simulink model "simulation model"  (R2022b)
settings: Solver=VariableStepAuto  StartTime=0.0  StopTime=2  RelTol=1e-3
undefined symbols (not defined in the file): a_prop, ACCtime, alfa, alfaPRO, Ba, Bf, Bp, Bv, IPR, matrixA, Ng_safe, No_perf, No_safe, Np, Np_safe, optimal_rotation, P3tDIVP2t_perf, P3tDIVP2t_safe, Q, Q_safe, T45_perf, T45_safe, Wf, xfuel, xlin, y, Yangle
libraries: fl_lib x31, nesl_utility x15, sh_lib x14, simulink x7, slpidlib x4, SimscapeFluids_lib x3
(part 2 of 2)

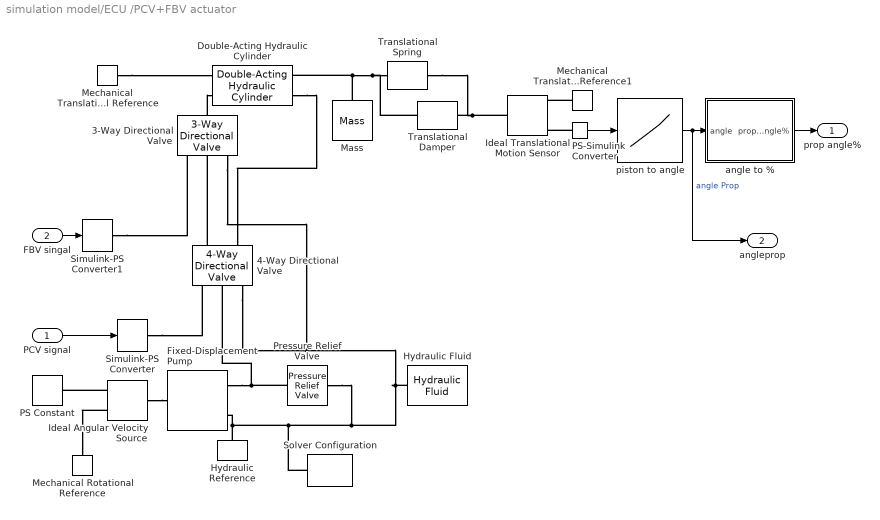
== system simulation model/ECU /PCV+FBV actuator ==
  PCV signal : Inport
  FBV singal : Inport  Port=2
  3-Way Directional Valve : sh_lib/Valves/Directional Valves/3-Way Directional Valve  area_spec=sh.valves.directional_valves.enum.area_spec.identical  mdl_type_identical=sh.valves.directional_valves.enum.mdl_type.linear  mdl_type_different=sh.valves.directional_valves.enum.mdl_type.linear  interp_method_identical=sh.valves.directional_valves.enum.interp_method.linear  interp_method_different=sh.valves.directional_valves.enum.interp_method.linear  extrap_method_identical=sh.valves.directional_valves.enum.extrap_method.linear  extrap_method_different=sh.valves.directional_valves.enum.extrap_method.linear  A_leak=1e-12 m^2  C_d=0.7  lam_spec=sh.valves.directional_valves.enum.lam_spec.pressure_ratio  B_lam=0.999  Re_cr=12  opening_max=1 m  area_max=0.05 m^2  opening_max_P_A=0.005 m  area_max_P_A=0.5e-4 m^2  opening_max_A_T=0.005 m  area_max_A_T=0.5e-4 m^2  opening_area_tab=[-.002, 0, .002, .005, .015] m  area_tab=[1e-09, 2.0352e-07, 4.0736e-05, .00011438, .00034356] m^2  opening_flow_rate_tab=[-.002, 0, .002, .005, .015] m  pressure_tab=[-10000000, -5000000, -2000000, 2000000, 5000000, 10000000] Pa  flow_rate_tab=[-1e-07, -7.0711e-08, -4.4721e-08, 4.4721e-08, 7.0711e-08, 1e-07; -2.0352e-05, -1.4391e-05, -9.1017e-06, 9.1017e-06, 1.4391e-05, 2.0352e-05; -.0040736, -.0028805, -.0018218, .0018218, .0028805, .0040736; -.011438, -.0080879, -.0051152, .0051152, .0080879, .011438; -.034356, -.024293, -.015364, .015364, .024293, .034356] m^3/s  opening_area_tab_P_A=[-.002, 0, .002, .005, .015] m  area_tab_P_A=[1e-09, 2.0352e-07, 4.0736e-05, .00011438, .00034356] m^2  opening_flow_rate_tab_P_A=[-.002, 0, .002, .005, .015] m  pressure_tab_P_A=[-10000000, -5000000, -2000000, 2000000, 5000000, 10000000] Pa  flow_rate_tab_P_A=[-1e-07, -7.0711e-08, -4.4721e-08, 4.4721e-08, 7.0711e-08, 1e-07; -2.0352e-05, -1.4391e-05, -9.1017e-06, 9.1017e-06, 1.4391e-05, 2.0352e-05; -.0040736, -.0028805, -.0018218, .0018218, .0028805, .0040736; -.011438, -.0080879, -.0051152, .0051152, .0080879, .011438; -.034356, -.024293, -.015364, .015364, .024293, .034356] m^3/s  opening_area_tab_A_T=[-.002, 0, .002, .005, .015] m  area_tab_A_T=[1e-09, 2.0352e-07, 4.0736e-05, .00011438, .00034356] m^2  opening_flow_rate_tab_A_T=[-.002, 0, .002, .005, .015] m  pressure_tab_A_T=[-10000000, -5000000, -2000000, 2000000, 5000000, 10000000] Pa  flow_rate_tab_A_T=[-1e-07, -7.0711e-08, -4.4721e-08, 4.4721e-08, 7.0711e-08, 1e-07; -2.0352e-05, -1.4391e-05, -9.1017e-06, 9.1017e-06, 1.4391e-05, 2.0352e-05; -.0040736, -.0028805, -.0018218, .0018218, .0028805, .0040736; -.011438, -.0080879, -.0051152, .0051152, .0080879, .011438; -.034356, -.024293, -.015364, .015364, .024293, .034356] m^3/s  x_0_P=0 m  x_0_T=0 m
      settings: InternalSimscapePortConfiguration="{\"Bottom\":[],\"Left\":[{\"id\":\"A\",\"label\":\"A\",\"type\":\"foundation.hydraulic.hydraulic\"}],\"Right\":[{\"id\":\"S\",\"label\":\"S\",\"type\":\"input\"},{\"id\":\"P\",\"label\":\"P\",\"type\":\"foundation.hydraulic.hydraulic\"},{\"id\":\"T\",\"label\":\"T\",\"type\":\"foundation.hydraulic.hydraulic\"}],\"Top\":[]}"
  4-Way Directional Valve : sh_lib/Valves/Directional Valves/4-Way Directional Valve  area_spec=sh.valves.directional_valves.enum.area_spec.identical  mdl_type_identical=sh.valves.directional_valves.enum.mdl_type.linear  mdl_type_different=sh.valves.directional_valves.enum.mdl_type.linear  interp_method_identical=sh.valves.directional_valves.enum.interp_method.linear  interp_method_different=sh.valves.directional_valves.enum.interp_method.linear  extrap_method_identical=sh.valves.directional_valves.enum.extrap_method.linear  extrap_method_different=sh.valves.directional_valves.enum.extrap_method.linear  A_leak=1e-12 m^2  C_d=0.7  lam_spec=sh.valves.directional_valves.enum.lam_spec.pressure_ratio  B_lam=0.999  Re_cr=12  opening_max=10 m  area_max=0.005 m^2  opening_max_P_A=0.005 m  area_max_P_A=0.5e-4 m^2  opening_max_P_B=0.005 m  area_max_P_B=0.5e-4 m^2  opening_max_A_T=0.005 m  area_max_A_T=0.5e-4 m^2  opening_max_B_T=0.005 m  area_max_B_T=0.5e-4 m^2  opening_area_tab=[-.002, 0, .002, .005, .015] m  area_tab=[1e-09, 2.0352e-07, 4.0736e-05, .00011438, .00034356] m^2  opening_flow_rate_tab=[-.002, 0, .002, .005, .015] m  pressure_tab=[-10000000, -5000000, -2000000, 2000000, 5000000, 10000000] Pa  flow_rate_tab=[-1e-07, -7.0711e-08, -4.4721e-08, 4.4721e-08, 7.0711e-08, 1e-07; -2.0352e-05, -1.4391e-05, -9.1017e-06, 9.1017e-06, 1.4391e-05, 2.0352e-05; -.0040736, -.0028805, -.0018218, .0018218, .0028805, .0040736; -.011438, -.0080879, -.0051152, .0051152, .0080879, .011438; -.034356, -.024293, -.015364, .015364, .024293, .034356] m^3/s  opening_area_tab_P_A=[-.002, 0, .002, .005, .015] m  area_tab_P_A=[1e-09, 2.0352e-07, 4.0736e-05, .00011438, .00034356] m^2  opening_flow_rate_tab_P_A=[-.002, 0, .002, .005, .015] m  pressure_tab_P_A=[-10000000, -5000000, -2000000, 2000000, 5000000, 10000000] Pa  flow_rate_tab_P_A=[-1e-07, -7.0711e-08, -4.4721e-08, 4.4721e-08, 7.0711e-08, 1e-07; -2.0352e-05, -1.4391e-05, -9.1017e-06, 9.1017e-06, 1.4391e-05, 2.0352e-05; -.0040736, -.0028805, -.0018218, .0018218, .0028805, .0040736; -.011438, -.0080879, -.0051152, .0051152, .0080879, .011438; -.034356, -.024293, -.015364, .015364, .024293, .034356] m^3/s  opening_area_tab_P_B=[-.002, 0, .002, .005, .015] m  area_tab_P_B=[1e-09, 2.0352e-07, 4.0736e-05, .00011438, .00034356] m^2  opening_flow_rate_tab_P_B=[-.002, 0, .002, .005, .015] m  pressure_tab_P_B=[-10000000, -5000000, -2000000, 2000000, 5000000, 10000000] Pa  flow_rate_tab_P_B=[-1e-07, -7.0711e-08, -4.4721e-08, 4.4721e-08, 7.0711e-08, 1e-07; -2.0352e-05, -1.4391e-05, -9.1017e-06, 9.1017e-06, 1.4391e-05, 2.0352e-05; -.0040736, -.0028805, -.0018218, .0018218, .0028805, .0040736; -.011438, -.0080879, -.0051152, .0051152, .0080879, .011438; -.034356, -.024293, -.015364, .015364, .024293, .034356] m^3/s  opening_area_tab_A_T=[-.002, 0, .002, .005, .015] m  area_tab_A_T=[1e-09, 2.0352e-07, 4.0736e-05, .00011438, .00034356] m^2  opening_flow_rate_tab_A_T=[-.002, 0, .002, .005, .015] m  pressure_tab_A_T=[-10000000, -5000000, -2000000, 2000000, 5000000, 10000000] Pa  flow_rate_tab_A_T=[-1e-07, -7.0711e-08, -4.4721e-08, 4.4721e-08, 7.0711e-08, 1e-07; -2.0352e-05, -1.4391e-05, -9.1017e-06, 9.1017e-06, 1.4391e-05, 2.0352e-05; -.0040736, -.0028805, -.0018218, .0018218, .0028805, .0040736; -.011438, -.0080879, -.0051152, .0051152, .0080879, .011438; -.034356, -.024293, -.015364, .015364, .024293, .034356] m^3/s  opening_area_tab_B_T=[-.002, 0, .002, .005, .015] m  area_tab_B_T=[1e-09, 2.0352e-07, 4.0736e-05, .00011438, .00034356] m^2  opening_flow_rate_tab_B_T=[-.002, 0, .002, .005, .015] m  pressure_tab_B_T=[-10000000, -5000000, -2000000, 2000000, 5000000, 10000000] Pa  flow_rate_tab_B_T=[-1e-07, -7.0711e-08, -4.4721e-08, 4.4721e-08, 7.0711e-08, 1e-07; -2.0352e-05, -1.4391e-05, -9.1017e-06, 9.1017e-06, 1.4391e-05, 2.0352e-05; -.0040736, -.0028805, -.0018218, .0018218, .0028805, .0040736; -.011438, -.0080879, -.0051152, .0051152, .0080879, .011438; -.034356, -.024293, -.015364, .015364, .024293, .034356] m^3/s  x_0_P_A=0 m  x_0_P_B=0 m  x_0_A_T=0 m  x_0_B_T=0 m
      settings: InternalSimscapePortConfiguration="{\"Bottom\":[],\"Left\":[{\"id\":\"A\",\"label\":\"A\",\"type\":\"foundation.hydraulic.hydraulic\"},{\"id\":\"B\",\"label\":\"B\",\"type\":\"foundation.hydraulic.hydraulic\"}],\"Right\":[{\"id\":\"S\",\"label\":\"S\",\"type\":\"input\"},{\"id\":\"P\",\"label\":\"P\",\"type\":\"foundation.hydraulic.hydraulic\"},{\"id\":\"T\",\"label\":\"T\",\"type\":\"foundation.hydraulic.hydraulic\"}],\"Top\":[]}"
  Double-Acting Hydraulic Cylinder : sh_lib/Hydraulic Cylinders/Double-Acting Hydraulic Cylinder  area_A=1e-3 m^2  area_B=0.5e-3 m^2  stroke=0.35 m  dead_vol_A=1e-4 m^3  dead_vol_B=1e-4 m^3  k_sh=1.4  or=sh.cylinders.enum.MechOrientationTranslational.Positive  stiff=1e6 N/m  D=150 N*s/m  hardstop_model=1  transition=0.1 mm  displacement_spec=foundation.enum.DisplacementSpec.Calculate  init_pos=0.215 m  init_pressure_A=0 Pa  init_pressure_B=0 Pa
      settings: LogSimulationData=on  InternalSimscapePortConfiguration="{\"Bottom\":[],\"Left\":[{\"id\":\"C\",\"label\":\"C\",\"type\":\"foundation.mechanical.translational.translational\"},{\"id\":\"A\",\"label\":\"A\",\"type\":\"foundation.hydraulic.hydraulic\"}],\"Right\":[{\"id\":\"R\",\"label\":\"R\",\"type\":\"foundation.mechanical.translational.translational\"},{\"id\":\"B\",\"label\":\"B\",\"type\":\"foundation.hydraulic.hydraulic\"}],\"Top\":[]}"
  Fixed-Displacement Pump : sh_lib/Pumps and Motors/Fixed-Displacement Pump  D=30 cm^3/rev  loss_spec=1  w_nominal=188 rad/s  pr_nominal=100e6 Pa  visc_nominal=18 cSt  dens_nominal=900 kg/m^3  efficiency_vol=0.92  no_load_torque=0.05 N*m  torque_pressure_coeff=0.6e-6 N*m/Pa  p_diff_eff_TLU=[100000, 1000000, 2000000] Pa  omega_eff_TLU=[25, 50, 100, 200, 300, 400] rad/s  vol_eff_TLU=[.816, .908, .954, .977, .981, .984; .325, .663, .831, .916, .925, .946; .137, .568, .78, .892, .893, .91]  mech_eff_TLU=[.996, .996, .996, .996, .996, .996; .988, .989, .989, .989, .989, .99; .981, .981, .982, .982, .983, .984]  p_diff_loss_TLU=[100000, 1000000, 2000000] Pa  omega_loss_TLU=[25, 50, 100, 200, 300, 400] rad/s  vol_loss_TLU=[.023, .023, .023, .023, .0285, .032; .0844, .0842, .0845, .084, .1125, .108; .1079, .108, .11, .108, .1605, .18] * 1e-3 m^3/s  mech_loss_TLU=[.002, .002, .002, .002, .002, .002; .0607, .0556, .0556, .0556, .0556, .0505; .1937, .1937, .1833, .1833, .1729, .1626] N*m  pressure_threshold=1e5 Pa  omega_threshold=10 rad/s  quadrant_check=0  pressure_check=0  min_valid_pressure=0 Pa  vol_eff_min=1e-3  vol_eff_max=1  mech_eff_min=1e-3  mech_eff_max=1
      settings: InternalSimscapePortConfiguration="{\"Bottom\":[],\"Left\":[{\"id\":\"S\",\"label\":\"S\",\"type\":\"foundation.mechanical.rotational.rotational\"}],\"Right\":[{\"id\":\"P\",\"label\":\"P\",\"type\":\"foundation.hydraulic.hydraulic\"},{\"id\":\"T\",\"label\":\"T\",\"type\":\"foundation.hydraulic.hydraulic\"}],\"Top\":[]}"
  Hydraulic Fluid : sh_lib/Hydraulic Utilities/Hydraulic Fluid  SelFluid=1  SysTemp=60  TrapAir=0.005  ViscDerFactor=1  range_error=2
  Hydraulic Reference : fl_lib/Hydraulic/Hydraulic Elements/Hydraulic Reference
  Ideal Angular Velocity Source : fl_lib/Mechanical/Mechanical Sources/Ideal Angular Velocity Source
  Ideal Translational Motion Sensor : fl_lib/Mechanical/Mechanical Sensors/Ideal Translational Motion Sensor  reference=foundation.enum.MeasurementReference.difference  acceleration_port=false  velocity_port=true  position_port=true  offset=0.215 m
  Mass : fl_lib/Mechanical/Translational Elements/Mass  mass=1000 kg  num_ports=foundation.enum.numPorts2.one  v_specify=off  v_priority=High  v=0 m/s  v_nominal_specify=off  v_nominal_unit=m/s  v_nominal_value=1  f_specify=off  f_priority=None  f=0 N  f_nominal_specify=off  f_nominal_unit=N  f_nominal_value=1
  Mechanical Rotational Reference : fl_lib/Mechanical/Rotational Elements/Mechanical Rotational Reference
  Mechanical Translational Reference : fl_lib/Mechanical/Translational Elements/Mechanical Translational Reference
  Mechanical Translational Reference1 : fl_lib/Mechanical/Translational Elements/Mechanical Translational Reference
  PS Constant : fl_lib/Physical Signals/Sources/PS Constant  constant=10
  PS-Simulink Converter : nesl_utility/PS-Simulink Converter  PhysicalDomain=network_engine_domain  SubClassName=ps_output  LeftPortType=input  RightPortType=output  PseudoPeriodic=off  Frequencies=[]  VectorFormat=inherit  Unit=inherit  AffineConversion=off
  Pressure Relief Valve : sh_lib/Valves/Pressure Control Valves/Pressure Relief Valve  valve_area_spec=1  p_diff_TLU=[30.15e5 : 15e3 : 31.35e5] Pa  area_TLU=[1 : 1 : 9] .* 1e-5 m^2  area_max=1e-4 m^2  pres_set=50e5 Pa  reg_range=5e5 Pa  C_d=0.7  A_leak=1e-12 m^2  lam_spec=1  B_lam=0.999  Re_cr=12  dynamic=0  tau=0.1 s  area_init=1e-12 m^2
      settings: InternalSimscapePortConfiguration="{\"Bottom\":[],\"Left\":[{\"id\":\"A\",\"label\":\"A\",\"type\":\"foundation.hydraulic.hydraulic\"}],\"Right\":[{\"id\":\"B\",\"label\":\"B\",\"type\":\"foundation.hydraulic.hydraulic\"}],\"Top\":[]}"
  Simulink-PS Converter : nesl_utility/Simulink-PS Converter  PhysicalDomain=network_engine_domain  SubClassName=ps_input  LeftPortType=input  RightPortType=output  PseudoPeriodic=off  Frequencies=[]  NoiseDistribution=none  NoiseParameters=[]  Unit=m  AffineConversion=on  FilteringAndDerivatives=provide  SimscapeFilterOrder=1  InputFilterTimeConstant=0.001  UdotUserProvided=0
  Simulink-PS Converter1 : nesl_utility/Simulink-PS Converter  PhysicalDomain=network_engine_domain  SubClassName=ps_input  LeftPortType=input  RightPortType=output  PseudoPeriodic=off  Frequencies=[]  NoiseDistribution=none  NoiseParameters=[]  Unit=m  AffineConversion=on  FilteringAndDerivatives=provide  SimscapeFilterOrder=1  InputFilterTimeConstant=0.001  UdotUserProvided=0
  Solver Configuration : nesl_utility/Solver Configuration  PhysicalDomain=network_engine_domain  SubClassName=solver  LeftPortType=input  RightPortType=generic  Tones=[]  Harmonics=[]  SimulateNoise=off  Profile=off  UseLocalSampling=off  EnableSwitchedLinearOptims=on  FrequencyDomain=off  UseCCode=off  RelTol=0.001  AbsTol=0.001  MinStep=1e-09  ToWorkspace=off  RevertToSquareIcSolve=off  NumHomotopyIterations=100  PhasorMode=off  PhasorModeNumHarmonics=1  ConsistencySolver=NEWTON_XTOL_AFTER_FTOL  IndexReductionMethod=DerivativeReplacement  DoDC=off  ResidualTolerance=1e-09  ConsistencyTolSource=GLOBAL  ConsistencyAbsTol=0.001  ConsistencyRelTol=0.001  ConsistencyTolFactor=0.001  UseLocalSolver=off  LocalSolverChoice=NE_BACKWARD_EULER_ADVANCER  ResolveIndetEquations=on  FunctionEvalNumThread=1  LocalSolverSampleTime=0.001  DoFixedCost=off  MaxNonlinIter=3  MaxModeIter=2  ComputeImpulses=off  ImpulseIterations=2  LinearAlgebra=auto  LinearAlgebraNumThread=0  EquationFormulation=NE_TIME_EF  DelaysMemoryBudget=1024  AutomaticFiltering=on  FilteringTimeConstant=0.001  PartitionStorageMethod=AS_NEEDED  PartitionMemoryBudget=1024  PartitionMethod=ROBUST
  Translational Damper : fl_lib/Mechanical/Translational Elements/Translational Damper  D=100000 N*s/m  v_specify=off  v_priority=None  v=0 m/s  v_nominal_specify=off  v_nominal_unit=m/s  v_nominal_value=1  f_specify=off  f_priority=None  f=0 N  f_nominal_specify=off  f_nominal_unit=N  f_nominal_value=1
  Translational Spring : fl_lib/Mechanical/Translational Elements/Translational Spring  spr_rate=1000 N/m  v_specify=off  v_priority=None  v=0 m/s  v_nominal_specify=off  v_nominal_unit=m/s  v_nominal_value=1  f_specify=off  f_priority=None  f=0 N  f_nominal_specify=off  f_nominal_unit=N  f_nominal_value=1  x_specify=off  x_priority=High  x=0 m  x_nominal_specify=off  x_nominal_unit=m  x_nominal_value=1
  angle to % : Subsystem
  piston to angle : Lookup_n-D  NumberOfTableDimensions=1  BreakpointsForDimension1=xlin  Table=alfaPRO  InternalRulePriority=Speed  RndMeth=Simplest
  prop angle% : Outport
  angleprop : Outport  Port=2
  wires:
  PS-Simulink Converter/1 -> piston to angle/1
  angle to %/1(prop angle%) -> prop angle%/1
  FBV singal/1 -> Simulink-PS Converter1/1
  PCV signal/1 -> Simulink-PS Converter/1
  piston to angle/1 -> angleprop/1, angle to %/1(angle)  "angle Prop"
  connections:
  Hydraulic Fluid/RConn1 -- 4-Way Directional Valve/RConn3 -- 3-Way Directional Valve/RConn3 -- Pressure Relief Valve/RConn1 -- Solver Configuration/RConn1 -- Fixed-Displacement Pump/RConn2 -- Hydraulic Reference/LConn1
  Fixed-Displacement Pump/RConn1 -- Pressure Relief Valve/LConn1 -- 4-Way Directional Valve/RConn2
  Mass/LConn1 -- Double-Acting Hydraulic Cylinder/RConn1 -- Translational Spring/LConn1 -- Translational Damper/LConn1
  Translational Spring/RConn1 -- Translational Damper/RConn1 -- Ideal Translational Motion Sensor/LConn1
  Mechanical Translational Reference1/LConn1 -- Ideal Translational Motion Sensor/RConn1
  PS-Simulink Converter/LConn1 -- Ideal Translational Motion Sensor/RConn3
  Mechanical Translational Reference/LConn1 -- Double-Acting Hydraulic Cylinder/LConn1
  Ideal Angular Velocity Source/LConn1 -- Fixed-Displacement Pump/LConn1
  Ideal Angular Velocity Source/RConn2 -- Mechanical Rotational Reference/LConn1
  Double-Acting Hydraulic Cylinder/RConn2 -- 4-Way Directional Valve/LConn2
  Simulink-PS Converter/RConn1 -- 4-Way Directional Valve/RConn1
  Ideal Angular Velocity Source/RConn1 -- PS Constant/RConn1
  4-Way Directional Valve/LConn1 -- 3-Way Directional Valve/RConn2
  3-Way Directional Valve/LConn1 -- Double-Acting Hydraulic Cylinder/LConn2
  Simulink-PS Converter1/RConn1 -- 3-Way Directional Valve/RConn1

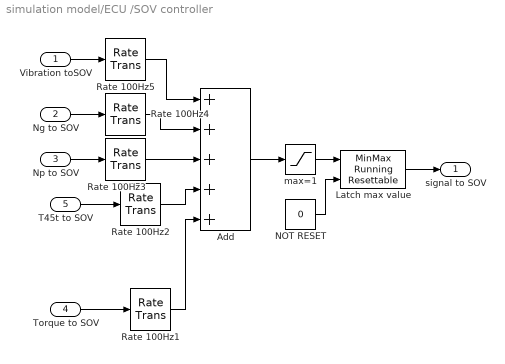
== system simulation model/ECU /SOV controller ==
  Vibration toSOV : Inport
  Ng to SOV : Inport  Port=2
  Np to SOV : Inport  Port=3
  Torque to SOV : Inport  Port=4
  T45t to SOV : Inport  Port=5
  Add : Sum  Inputs=+++++  OutMax=[1]
  Latch max value : simulink/Math Operations/MinMax Running Resettable  Function=max  vinit=0.0
  NOT RESET : Constant  Value=0
  Rate 100Hz{1..5} (5 alike) : RateTransition  OutPortSampleTimeMultiple=2  OutPortSampleTime=0.01
  max=1 : Saturate  UpperLimit=1  LowerLimit=0
  signal to SOV : Outport
  wires:
  Vibration toSOV/1 -> Rate 100Hz5/1
  Ng to SOV/1 -> Rate 100Hz4/1
  Np to SOV/1 -> Rate 100Hz3/1
  T45t to SOV/1 -> Rate 100Hz2/1
  Torque to SOV/1 -> Rate 100Hz1/1
  NOT RESET/1 -> Latch max value/2
  max=1/1 -> Latch max value/1
  Add/1 -> max=1/1
  Latch max value/1 -> signal to SOV/1
  Rate 100Hz1/1 -> Add/5
  Rate 100Hz2/1 -> Add/4
  Rate 100Hz3/1 -> Add/3
  Rate 100Hz4/1 -> Add/2
  Rate 100Hz5/1 -> Add/1

== system simulation model/ECU /T1 sensor ==
  T1 : Inport
  Add : Sum
  Add1 : Sum
  Bus Creator : BusCreator  Inputs=2
  Delay : Delay  DelayLength=25  InitialCondition=1  SampleTime=0.001
  Normal Noise : RandomNumber  Variance=((0.01)^2)*pi/2  Seed=41  SampleTime=0.2
  Normal Noise1 : RandomNumber  Variance=((0.01)^2)*pi/2  Seed=42  SampleTime=0.2
  Product : Product
  Product1 : Product
  Rate 5Hz : RateTransition  OutPortSampleTimeMultiple=2  OutPortSampleTime=0.2
  T1sen : Outport
  wires:
  Normal Noise1/1 -> Product1/2
  Normal Noise/1 -> Product/2
  Add1/1 -> Bus Creator/2
  Bus Creator/1 -> T1sen/1
  Rate 5Hz/1 -> Add/1, Product/1, Add1/1, Product1/1
  Add/1 -> Bus Creator/1
  Product1/1 -> Add1/2
  Product/1 -> Add/2
  Delay/1 -> Rate 5Hz/1
  T1/1 -> Delay/1

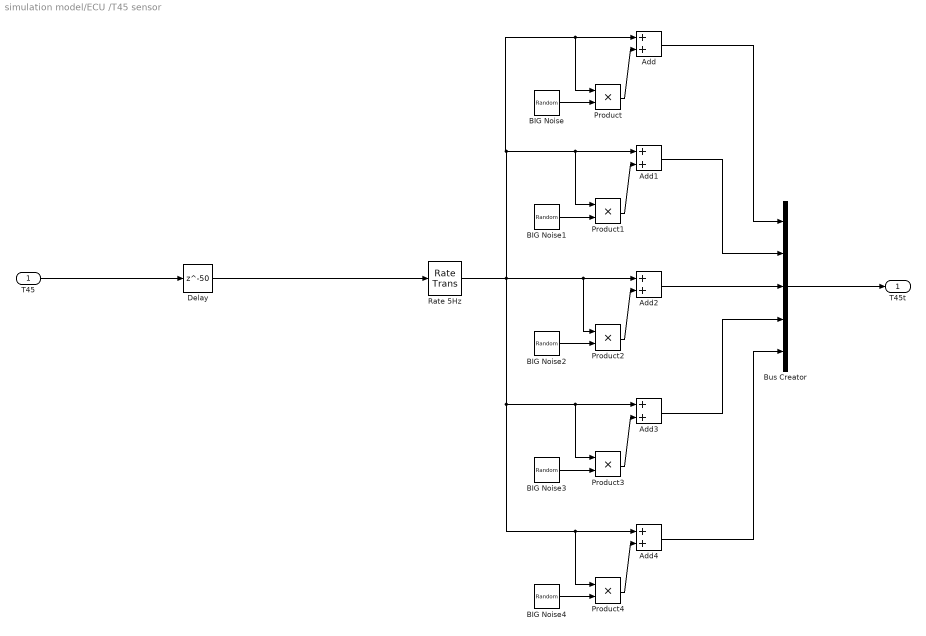
== system simulation model/ECU /T45 sensor ==
  T45 : Inport
  Add{,1..4} (5 alike) : Sum
  BIG Noise : RandomNumber  Variance=((0.015)^2)*pi/2  Seed=51  SampleTime=0.2
  BIG Noise1 : RandomNumber  Variance=((0.015)^2)*pi/2  Seed=53  SampleTime=0.2
  BIG Noise2 : RandomNumber  Variance=((0.015)^2)*pi/2  Seed=55  SampleTime=0.2
  BIG Noise3 : RandomNumber  Variance=((0.015)^2)*pi/2  Seed=57  SampleTime=0.2
  BIG Noise4 : RandomNumber  Variance=((0.015)^2)*pi/2  Seed=59  SampleTime=0.2
  Bus Creator : BusCreator  Inputs=5
  Delay : Delay  DelayLength=50  InitialCondition=1  SampleTime=0.001
  Product{,1..4} (5 alike) : Product
  Rate 5Hz : RateTransition  OutPortSampleTime=0.2
  T45t : Outport
  wires:
  BIG Noise/1 -> Product/2
  Product/1 -> Add/2
  Product1/1 -> Add1/2
  BIG Noise1/1 -> Product1/2
  Product2/1 -> Add2/2
  BIG Noise2/1 -> Product2/2
  Product3/1 -> Add3/2
  BIG Noise3/1 -> Product3/2
  Product4/1 -> Add4/2
  Rate 5Hz/1 -> Add/1, Product/1, Add1/1, Product1/1, Product2/1, Add2/1, Add3/1, Product3/1, Add4/1, Product4/1
  BIG Noise4/1 -> Product4/2
  Bus Creator/1 -> T45t/1
  Add2/1 -> Bus Creator/3
  Add3/1 -> Bus Creator/4
  Add4/1 -> Bus Creator/5
  Add1/1 -> Bus Creator/2
  Add/1 -> Bus Creator/1
  T45/1 -> Delay/1
  Delay/1 -> Rate 5Hz/1

== system simulation model/ECU /T45t limiter ==
  T45t : Inport
  Constant2 : Constant  Value=-1
  Constant3 : Constant
  Safe switch : Subsystem
  Subtract : Sum  Inputs=+-
  Switch1 : Switch  Criteria=u2 > Threshold  Threshold=T45_safe  SaturateOnIntegerOverflow=off  InputSameDT=off
  T45 VOTER : MATLAB Function  TreatAsAtomicUnit=on
  Torque_performance : Constant  Value=T45_perf
  T45t to SOV : Outport
  T45t to FMV : Outport  Port=2
  wires:
  Subtract/1 -> T45t to FMV/1
  ? -> ?
  Switch1/1 -> Safe switch/1(In1)
  Constant2/1 -> Switch1/3
  Constant3/1 -> Switch1/1
  Torque_performance/1 -> Subtract/2
  T45 VOTER/1(y) -> Subtract/1, Switch1/2
  T45t/1 -> T45 VOTER/1(u)
  Safe switch/1(T45t to SOV) -> T45t to SOV/1

== system simulation model/ECU /Torque limiters ==
  Torque sen : Inport
  Add : Sum
  Constant : Constant  Value=-1
  Constant1 : Constant
  Demux : Demux  Outputs=2
  Gain : Gain  Gain=0.5
  Safe switch : Subsystem
  Switch : Switch  Criteria=u2 > Threshold  Threshold=Q_safe  SaturateOnIntegerOverflow=off  InputSameDT=off
  Torque to SOV : Outport
  wires:
  Gain/1 -> Switch/2
  Constant1/1 -> Switch/1
  Torque sen/1 -> Demux/1
  Constant/1 -> Switch/3
  Demux/2 -> Add/2
  Add/1 -> Gain/1
  Demux/1 -> Add/1
  Switch/1 -> Safe switch/1(In1)
  Safe switch/1(Torque to SOV) -> Torque to SOV/1

== system simulation model/ECU /Torque sensor ==
  Np : Inport
  Add : Sum
  Add1 : Sum
  Bus Creator : BusCreator  Inputs=2
  Gain : Gain  Gain=2
  Gain1 : Gain  Gain=2
  Normal Noise1 : RandomNumber  Variance=((0.017)^2)*pi/2  Seed=21  SampleTime=0.01
  Normal Noise2 : RandomNumber  Variance=((0.017)^2)*pi/2  Seed=23  SampleTime=0.01
  Np->Q : Lookup_n-D  NumberOfTableDimensions=1  BreakpointsForDimension1=Np  Table=Q  InternalRulePriority=Speed  RndMeth=Simplest
  Product : Product
  Product1 : Product
  Rate 100Hz : RateTransition  OutPortSampleTimeMultiple=2  OutPortSampleTime=0.01
  Torque sen : Outport
  wires:
  Normal Noise1/1 -> Gain/1
  Product/1 -> Add/2
  Gain/1 -> Product/2
  Normal Noise2/1 -> Gain1/1
  Product1/1 -> Add1/2
  Gain1/1 -> Product1/2
  Rate 100Hz/1 -> Add1/1, Product1/1, Add/1, Product/1
  Add1/1 -> Bus Creator/2
  Np/1 -> Np->Q/1
  Add/1 -> Bus Creator/1
  Bus Creator/1 -> Torque sen/1
  Np->Q/1 -> Rate 100Hz/1

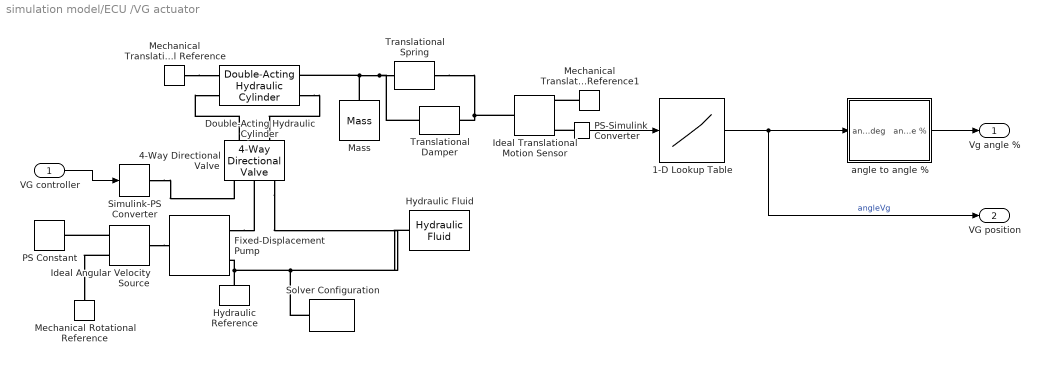
== system simulation model/ECU /VG actuator ==
  VG controller : Inport
  1-D Lookup Table : Lookup_n-D  NumberOfTableDimensions=1  BreakpointsForDimension1=Yangle  Table=alfa  InternalRulePriority=Speed  RndMeth=Simplest
  4-Way Directional Valve : sh_lib/Valves/Directional Valves/4-Way Directional Valve  area_spec=sh.valves.directional_valves.enum.area_spec.identical  mdl_type_identical=sh.valves.directional_valves.enum.mdl_type.linear  mdl_type_different=sh.valves.directional_valves.enum.mdl_type.linear  interp_method_identical=sh.valves.directional_valves.enum.interp_method.linear  interp_method_different=sh.valves.directional_valves.enum.interp_method.linear  extrap_method_identical=sh.valves.directional_valves.enum.extrap_method.linear  extrap_method_different=sh.valves.directional_valves.enum.extrap_method.linear  A_leak=1e-12 m^2  C_d=20  lam_spec=sh.valves.directional_valves.enum.lam_spec.pressure_ratio  B_lam=0.999  Re_cr=12  opening_max=0.005 m  area_max=0.5e-2 m^2  opening_max_P_A=0.005 m  area_max_P_A=0.5e-4 m^2  opening_max_P_B=0.005 m  area_max_P_B=0.5e-4 m^2  opening_max_A_T=0.005 m  area_max_A_T=0.5e-4 m^2  opening_max_B_T=0.005 m  area_max_B_T=0.5e-4 m^2  opening_area_tab=[-.002, 0, .002, .005, .015] m  area_tab=[1e-09, 2.0352e-07, 4.0736e-05, .00011438, .00034356] m^2  opening_flow_rate_tab=[-.002, 0, .002, .005, .015] m  pressure_tab=[-10000000, -5000000, -2000000, 2000000, 5000000, 10000000] Pa  flow_rate_tab=[-1e-07, -7.0711e-08, -4.4721e-08, 4.4721e-08, 7.0711e-08, 1e-07; -2.0352e-05, -1.4391e-05, -9.1017e-06, 9.1017e-06, 1.4391e-05, 2.0352e-05; -.0040736, -.0028805, -.0018218, .0018218, .0028805, .0040736; -.011438, -.0080879, -.0051152, .0051152, .0080879, .011438; -.034356, -.024293, -.015364, .015364, .024293, .034356] m^3/s  opening_area_tab_P_A=[-.002, 0, .002, .005, .015] m  area_tab_P_A=[1e-09, 2.0352e-07, 4.0736e-05, .00011438, .00034356] m^2  opening_flow_rate_tab_P_A=[-.002, 0, .002, .005, .015] m  pressure_tab_P_A=[-10000000, -5000000, -2000000, 2000000, 5000000, 10000000] Pa  flow_rate_tab_P_A=[-1e-07, -7.0711e-08, -4.4721e-08, 4.4721e-08, 7.0711e-08, 1e-07; -2.0352e-05, -1.4391e-05, -9.1017e-06, 9.1017e-06, 1.4391e-05, 2.0352e-05; -.0040736, -.0028805, -.0018218, .0018218, .0028805, .0040736; -.011438, -.0080879, -.0051152, .0051152, .0080879, .011438; -.034356, -.024293, -.015364, .015364, .024293, .034356] m^3/s  opening_area_tab_P_B=[-.002, 0, .002, .005, .015] m  area_tab_P_B=[1e-09, 2.0352e-07, 4.0736e-05, .00011438, .00034356] m^2  opening_flow_rate_tab_P_B=[-.002, 0, .002, .005, .015] m  pressure_tab_P_B=[-10000000, -5000000, -2000000, 2000000, 5000000, 10000000] Pa  flow_rate_tab_P_B=[-1e-07, -7.0711e-08, -4.4721e-08, 4.4721e-08, 7.0711e-08, 1e-07; -2.0352e-05, -1.4391e-05, -9.1017e-06, 9.1017e-06, 1.4391e-05, 2.0352e-05; -.0040736, -.0028805, -.0018218, .0018218, .0028805, .0040736; -.011438, -.0080879, -.0051152, .0051152, .0080879, .011438; -.034356, -.024293, -.015364, .015364, .024293, .034356] m^3/s  opening_area_tab_A_T=[-.002, 0, .002, .005, .015] m  area_tab_A_T=[1e-09, 2.0352e-07, 4.0736e-05, .00011438, .00034356] m^2  opening_flow_rate_tab_A_T=[-.002, 0, .002, .005, .015] m  pressure_tab_A_T=[-10000000, -5000000, -2000000, 2000000, 5000000, 10000000] Pa  flow_rate_tab_A_T=[-1e-07, -7.0711e-08, -4.4721e-08, 4.4721e-08, 7.0711e-08, 1e-07; -2.0352e-05, -1.4391e-05, -9.1017e-06, 9.1017e-06, 1.4391e-05, 2.0352e-05; -.0040736, -.0028805, -.0018218, .0018218, .0028805, .0040736; -.011438, -.0080879, -.0051152, .0051152, .0080879, .011438; -.034356, -.024293, -.015364, .015364, .024293, .034356] m^3/s  opening_area_tab_B_T=[-.002, 0, .002, .005, .015] m  area_tab_B_T=[1e-09, 2.0352e-07, 4.0736e-05, .00011438, .00034356] m^2  opening_flow_rate_tab_B_T=[-.002, 0, .002, .005, .015] m  pressure_tab_B_T=[-10000000, -5000000, -2000000, 2000000, 5000000, 10000000] Pa  flow_rate_tab_B_T=[-1e-07, -7.0711e-08, -4.4721e-08, 4.4721e-08, 7.0711e-08, 1e-07; -2.0352e-05, -1.4391e-05, -9.1017e-06, 9.1017e-06, 1.4391e-05, 2.0352e-05; -.0040736, -.0028805, -.0018218, .0018218, .0028805, .0040736; -.011438, -.0080879, -.0051152, .0051152, .0080879, .011438; -.034356, -.024293, -.015364, .015364, .024293, .034356] m^3/s  x_0_P_A=0 m  x_0_P_B=0 m  x_0_A_T=0 m  x_0_B_T=0 m
      settings: InternalSimscapePortConfiguration="{\"Bottom\":[],\"Left\":[{\"id\":\"A\",\"label\":\"A\",\"type\":\"foundation.hydraulic.hydraulic\"},{\"id\":\"B\",\"label\":\"B\",\"type\":\"foundation.hydraulic.hydraulic\"}],\"Right\":[{\"id\":\"S\",\"label\":\"S\",\"type\":\"input\"},{\"id\":\"P\",\"label\":\"P\",\"type\":\"foundation.hydraulic.hydraulic\"},{\"id\":\"T\",\"label\":\"T\",\"type\":\"foundation.hydraulic.hydraulic\"}],\"Top\":[]}"
  Double-Acting Hydraulic Cylinder : sh_lib/Hydraulic Cylinders/Double-Acting Hydraulic Cylinder  area_A=1e-3 m^2  area_B=1e-3 m^2  stroke=2 m  dead_vol_A=1e-4 m^3  dead_vol_B=1e-4 m^3  k_sh=1.4  or=sh.cylinders.enum.MechOrientationTranslational.Positive  stiff=1e6 N/m  D=150 N*s/m  hardstop_model=1  transition=0.1 mm  displacement_spec=foundation.enum.DisplacementSpec.Calculate  init_pos=1.5 m  init_pressure_A=0 Pa  init_pressure_B=0 Pa
      settings: LogSimulationData=on  InternalSimscapePortConfiguration="{\"Bottom\":[],\"Left\":[{\"id\":\"C\",\"label\":\"C\",\"type\":\"foundation.mechanical.translational.translational\"},{\"id\":\"A\",\"label\":\"A\",\"type\":\"foundation.hydraulic.hydraulic\"}],\"Right\":[{\"id\":\"R\",\"label\":\"R\",\"type\":\"foundation.mechanical.translational.translational\"},{\"id\":\"B\",\"label\":\"B\",\"type\":\"foundation.hydraulic.hydraulic\"}],\"Top\":[]}"
  Fixed-Displacement Pump : sh_lib/Pumps and Motors/Fixed-Displacement Pump  D=10 cm^3/rev  loss_spec=1  w_nominal=500 rad/s  pr_nominal=100e5 Pa  visc_nominal=18 cSt  dens_nominal=900 kg/m^3  efficiency_vol=0.92  no_load_torque=0.05 N*m  torque_pressure_coeff=0.6e-6 N*m/Pa  p_diff_eff_TLU=[100000, 1000000, 2000000] Pa  omega_eff_TLU=[25, 50, 100, 200, 300, 400] rad/s  vol_eff_TLU=[.816, .908, .954, .977, .981, .984; .325, .663, .831, .916, .925, .946; .137, .568, .78, .892, .893, .91]  mech_eff_TLU=[.996, .996, .996, .996, .996, .996; .988, .989, .989, .989, .989, .99; .981, .981, .982, .982, .983, .984]  p_diff_loss_TLU=[100000, 1000000, 2000000] Pa  omega_loss_TLU=[25, 50, 100, 200, 300, 400] rad/s  vol_loss_TLU=[.023, .023, .023, .023, .0285, .032; .0844, .0842, .0845, .084, .1125, .108; .1079, .108, .11, .108, .1605, .18] * 1e-3 m^3/s  mech_loss_TLU=[.002, .002, .002, .002, .002, .002; .0607, .0556, .0556, .0556, .0556, .0505; .1937, .1937, .1833, .1833, .1729, .1626] N*m  pressure_threshold=1e5 Pa  omega_threshold=10 rad/s  quadrant_check=0  pressure_check=0  min_valid_pressure=0 Pa  vol_eff_min=1e-3  vol_eff_max=1  mech_eff_min=1e-3  mech_eff_max=1
      settings: InternalSimscapePortConfiguration="{\"Bottom\":[],\"Left\":[{\"id\":\"S\",\"label\":\"S\",\"type\":\"foundation.mechanical.rotational.rotational\"}],\"Right\":[{\"id\":\"P\",\"label\":\"P\",\"type\":\"foundation.hydraulic.hydraulic\"},{\"id\":\"T\",\"label\":\"T\",\"type\":\"foundation.hydraulic.hydraulic\"}],\"Top\":[]}"
  Hydraulic Fluid : sh_lib/Hydraulic Utilities/Hydraulic Fluid  SelFluid=1  SysTemp=60  TrapAir=0.005  ViscDerFactor=1  range_error=2
  Hydraulic Reference : fl_lib/Hydraulic/Hydraulic Elements/Hydraulic Reference
  Ideal Angular Velocity Source : fl_lib/Mechanical/Mechanical Sources/Ideal Angular Velocity Source
  Ideal Translational Motion Sensor : fl_lib/Mechanical/Mechanical Sensors/Ideal Translational Motion Sensor  reference=foundation.enum.MeasurementReference.difference  acceleration_port=false  velocity_port=true  position_port=true  offset=1.5 m
  Mass : fl_lib/Mechanical/Translational Elements/Mass  mass=1 kg  num_ports=foundation.enum.numPorts2.one  v_specify=off  v_priority=High  v=0 m/s  v_nominal_specify=off  v_nominal_unit=m/s  v_nominal_value=1  f_specify=off  f_priority=None  f=0 N  f_nominal_specify=off  f_nominal_unit=N  f_nominal_value=1
  Mechanical Rotational Reference : fl_lib/Mechanical/Rotational Elements/Mechanical Rotational Reference
  Mechanical Translational Reference : fl_lib/Mechanical/Translational Elements/Mechanical Translational Reference
  Mechanical Translational Reference1 : fl_lib/Mechanical/Translational Elements/Mechanical Translational Reference
  PS Constant : fl_lib/Physical Signals/Sources/PS Constant  constant=20
  PS-Simulink Converter : nesl_utility/PS-Simulink Converter  PhysicalDomain=network_engine_domain  SubClassName=ps_output  LeftPortType=input  RightPortType=output  PseudoPeriodic=off  Frequencies=[]  VectorFormat=inherit  Unit=inherit  AffineConversion=off
  Simulink-PS Converter : nesl_utility/Simulink-PS Converter  PhysicalDomain=network_engine_domain  SubClassName=ps_input  LeftPortType=input  RightPortType=output  PseudoPeriodic=off  Frequencies=[]  NoiseDistribution=none  NoiseParameters=[]  Unit=m  AffineConversion=on  FilteringAndDerivatives=provide  SimscapeFilterOrder=1  InputFilterTimeConstant=0.001  UdotUserProvided=0
  Solver Configuration : nesl_utility/Solver Configuration  PhysicalDomain=network_engine_domain  SubClassName=solver  LeftPortType=input  RightPortType=generic  Tones=[]  Harmonics=[]  SimulateNoise=off  Profile=off  UseLocalSampling=off  EnableSwitchedLinearOptims=on  FrequencyDomain=off  UseCCode=off  RelTol=0.001  AbsTol=0.001  MinStep=1e-09  ToWorkspace=off  RevertToSquareIcSolve=off  NumHomotopyIterations=100  PhasorMode=off  PhasorModeNumHarmonics=1  ConsistencySolver=NEWTON_XTOL_AFTER_FTOL  IndexReductionMethod=DerivativeReplacement  DoDC=off  ResidualTolerance=1e-09  ConsistencyTolSource=GLOBAL  ConsistencyAbsTol=0.001  ConsistencyRelTol=0.001  ConsistencyTolFactor=0.001  UseLocalSolver=off  LocalSolverChoice=NE_BACKWARD_EULER_ADVANCER  ResolveIndetEquations=on  FunctionEvalNumThread=1  LocalSolverSampleTime=0.001  DoFixedCost=off  MaxNonlinIter=3  MaxModeIter=2  ComputeImpulses=off  ImpulseIterations=2  LinearAlgebra=auto  LinearAlgebraNumThread=0  EquationFormulation=NE_TIME_EF  DelaysMemoryBudget=1024  AutomaticFiltering=on  FilteringTimeConstant=0.001  PartitionStorageMethod=AS_NEEDED  PartitionMemoryBudget=1024  PartitionMethod=ROBUST
  Translational Damper : fl_lib/Mechanical/Translational Elements/Translational Damper  D=100 N*s/m  v_specify=off  v_priority=None  v=0 m/s  v_nominal_specify=off  v_nominal_unit=m/s  v_nominal_value=1  f_specify=off  f_priority=None  f=0 N  f_nominal_specify=off  f_nominal_unit=N  f_nominal_value=1
  Translational Spring : fl_lib/Mechanical/Translational Elements/Translational Spring  spr_rate=1 N/m  v_specify=off  v_priority=None  v=0 m/s  v_nominal_specify=off  v_nominal_unit=m/s  v_nominal_value=1  f_specify=off  f_priority=None  f=0 N  f_nominal_specify=off  f_nominal_unit=N  f_nominal_value=1  x_specify=off  x_priority=High  x=0 m  x_nominal_specify=off  x_nominal_unit=m  x_nominal_value=1
  angle to angle % : Subsystem
  Vg angle % : Outport
  VG position : Outport  Port=2
  wires:
  PS-Simulink Converter/1 -> 1-D Lookup Table/1
  1-D Lookup Table/1 -> VG position/1, angle to angle %/1(ange deg)  "angleVg"
  VG controller/1 -> Simulink-PS Converter/1
  angle to angle %/1(angle %) -> Vg angle %/1
  connections:
  Solver Configuration/RConn1 -- Fixed-Displacement Pump/RConn2 -- Hydraulic Reference/LConn1 -- Hydraulic Fluid/RConn1 -- 4-Way Directional Valve/RConn3
  Fixed-Displacement Pump/RConn1 -- 4-Way Directional Valve/RConn2
  Mass/LConn1 -- Double-Acting Hydraulic Cylinder/RConn1 -- Translational Spring/LConn1 -- Translational Damper/LConn1
  Translational Spring/RConn1 -- Translational Damper/RConn1 -- Ideal Translational Motion Sensor/LConn1
  Ideal Angular Velocity Source/RConn1 -- PS Constant/RConn1
  Double-Acting Hydraulic Cylinder/RConn2 -- 4-Way Directional Valve/LConn2
  Ideal Angular Velocity Source/RConn2 -- Mechanical Rotational Reference/LConn1
  Simulink-PS Converter/RConn1 -- 4-Way Directional Valve/RConn1
  Mechanical Translational Reference1/LConn1 -- Ideal Translational Motion Sensor/RConn1
  Mechanical Translational Reference/LConn1 -- Double-Acting Hydraulic Cylinder/LConn1
  4-Way Directional Valve/LConn1 -- Double-Acting Hydraulic Cylinder/LConn2
  Ideal Angular Velocity Source/LConn1 -- Fixed-Displacement Pump/LConn1
  PS-Simulink Converter/LConn1 -- Ideal Translational Motion Sensor/RConn3

== system simulation model/ECU /VG controler ==
  T1 : Inport
  feedback : Inport  Port=2
  1-D Lookup Table : Lookup_n-D  NumberOfTableDimensions=1  BreakpointsForDimension1=y  Table=alfa  InternalRulePriority=Speed  RndMeth=Simplest
  10 value average : Subsystem
  Add : Sum
  Demux : Demux  Outputs=2
  Gain : Gain  Gain=0.5
  IGV_error : Sum  Inputs=+-
  PID Controller : slpidlib/PID Controller  Controller=P  Form=Parallel  TimeDomain=Continuous-time  UseExternalTs=off  SampleTime=-1  IntegratorMethod=Forward Euler  FilterMethod=Forward Euler  ControllerParametersSource=internal  P=1  I=1  UseKiTs=off  D=0  N=100  UseFilter=on  TunerSelectOption=Transfer Function Based (PID Tuner App)  InitialConditionSource=internal  InitialConditionForIntegrator=0  InitialConditionForFilter=0  DifferentiatorICPrevScaledInput=0  ExternalReset=none  TrackingMode=off  Kt=1  LimitOutput=off  SatLimitsSource=internal  UpperSaturationLimit=inf  LowerSaturationLimit=-inf  LinearizeAsGain=on  AntiWindupMode=none  Kb=1  LimitIntegrator=off  UpperIntegratorSaturationLimit=inf  LowerIntegratorSaturationLimit=-inf  POutMin=[]  POutMax=[]  IOutMin=[]  IOutMax=[]  DOutMin=[]  DOutMax=[]  NOutMin=[]  NOutMax=[]  SumOutMin=[]  SumOutMax=[]  SaturationOutMin=[]  SaturationOutMax=[]  PParamMin=[]  PParamMax=[]  IParamMin=[]  IParamMax=[]  DParamMin=[]  DParamMax=[]  NParamMin=[]  NParamMax=[]  KbParamMin=[]  KbParamMax=[]  KtParamMin=[]  KtParamMax=[]  KbOutMin=[]  KbOutMax=[]  KtOutMin=[]  KtOutMax=[]  IntegratorOutMin=[]  IntegratorOutMax=[]  FilterOutMin=[]  FilterOutMax=[]  SumI1OutMin=[]  SumI1OutMax=[]  SumI2OutMin=[]  SumI2OutMax=[]  SumI3OutMin=[]  SumI3OutMax=[]  SumI4OutMin=[]  SumI4OutMax=[]  SumDOutMin=[]  SumDOutMax=[]  DifferentiatorOutMin=[]  DifferentiatorOutMax=[]  FilterDiffOutCoefMin=[]  FilterDiffOutCoefMax=[]  ReciprocalOutMin=[]  ReciprocalOutMax=[]  SumDenOutMin=[]  SumDenOutMax=[]  SumNumOutMin=[]  SumNumOutMax=[]  DivideOutMin=[]  DivideOutMax=[]  UdiffTsProdOutMin=[]  UdiffTsProdOutMax=[]  NTsProdOutMin=[]  NTsProdOutMax=[]  UintegralTsProdOutMin=[]  UintegralTsProdOutMax=[]  UngainTsProdOutMin=[]  UngainTsProdOutMax=[]  ClampingZeroOutDataTypeStr=Inherit: Inherit via back propagation  ClampingZeroOutMin=[]  ClampingZeroOutMax=[]  FilterDenConstantOutDataTypeStr=Inherit: Inherit via back propagation  FilterDenConstantOutMin=[]  FilterDenConstantOutMax=[]  PCopyOutDataTypeStr=Inherit: Inherit via back propagation  PCopyOutMin=[]  PCopyOutMax=[]  NCopyOutDataTypeStr=Inherit: Inherit via back propagation  NCopyOutMin=[]  NCopyOutMax=[]  IntegratorContinuousStateAttributes=''  IntegratorStateMustResolveToSignalObject=off  IntegratorRTWStateStorageClass=Auto  FilterContinuousStateAttributes=''  FilterStateMustResolveToSignalObject=off  FilterRTWStateStorageClass=Auto  ParallelPVariant=InternalParameters  IdealPVariant=Disabled  IVariant=Disabled  DVariant=Disabled  IntegratorVariant=Disabled  SatVariant=Disabled  AWVariant=Disabled  PCopyVariant=Disabled  TRVariant=Disabled  FdbkBlocksVariant=Forward  IdealPFdbkVariant=Disabled  SatFdbkVariant=Disabled  DerivativeFilterVariant=Disabled  NVariant=Disabled  NCopyVariant=Disabled_SignalSpec  FilterICVariant=Disabled  IntegratorICVariant=Disabled  ExternalResetVariant=Disabled  TRSumVariant=Passthrough  SumFdbkVariant=Disabled  SumVariant=Passthrough_P  TsampFilterVariant=InternalTs  TsampNgainVariant=Passthrough  TsampIntegralVariant=Disabled_SignalSpec  ExternalSaturationOutDataTypeStr=Inherit: Same as second input
  Rate Transition : RateTransition  OutPortSampleTime=0.1
  VG signal : Outport
  wires:
  1-D Lookup Table/1 -> IGV_error/1
  feedback/1 -> IGV_error/2
  IGV_error/1 -> 10 value average/1(Input)
  PID Controller/1 -> VG signal/1
  Demux/1 -> Add/1
  T1/1 -> Demux/1
  Add/1 -> Gain/1
  Demux/2 -> Add/2
  Gain/1 -> Rate Transition/1
  10 value average/1(Output) -> PID Controller/1
  Rate Transition/1 -> 1-D Lookup Table/1

== system simulation model/ECU /VG sensor ==
  VGact pos : Inport
  E2ECU : Inport  Port=2
  1% MAD : RandomNumber  Variance=((0.01)^2)*pi/2  Seed=2  SampleTime=0.01
  Add2 : Sum
  FAKE POSITION : Constant  Value=-20
  Product2 : Product
  Rate 100Hz : RateTransition  OutPortSampleTimeMultiple=2  OutPortSampleTime=0.01
  Switch : Switch  Criteria=u2 > Threshold  SaturateOnIntegerOverflow=off  InputSameDT=off
  VGact sens : Outport
  wires:
  Rate 100Hz/1 -> Add2/1, Product2/1
  Product2/1 -> Add2/2
  1% MAD/1 -> Product2/2
  Add2/1 -> Switch/3
  E2ECU/1 -> Switch/2
  FAKE POSITION/1 -> Switch/1
  VGact pos/1 -> Rate 100Hz/1
  Switch/1 -> VGact sens/1

== system simulation model/ECU /Vibration sensor ==
  emergency3 : Inport
  0.15 s Delay : Delay  DelayLength=20  SampleTime=0.01
  Vib to SOV : Outport
  wires:
  emergency3/1 -> 0.15 s Delay/1
  0.15 s Delay/1 -> Vib to SOV/1

== system simulation model/ESU/Main subsystem ==
  u : Inport
  A : Constant  Value=matrixA
  Integrator : Integrator  InitialCondition=1  LimitOutput=on  UpperSaturationLimit=2  LowerSaturationLimit=0
  MATLAB Function1 : MATLAB Function  TreatAsAtomicUnit=on
  Rate 100Hz : RateTransition  OutPortSampleTimeMultiple=2  OutPortSampleTime=0.1
  toECU : Outport
  wires:
  u/1 -> Rate 100Hz/1
  MATLAB Function1/1(y) -> Integrator/1
  Integrator/1 -> toECU/1
  A/1 -> MATLAB Function1/2(A)
  Rate 100Hz/1 -> MATLAB Function1/1(u)

== system simulation model/ESU/air bleed subsystem ==
  dp3 value : Inport
  Constant : Constant  Value=Ba
  Derivative : Derivative
  Product : Product
  Saturation : Saturate  UpperLimit=0.25  LowerLimit=-0.25
  Dp3a : Outport
  wires:
  Product/1 -> Dp3a/1
  Derivative/1 -> Saturation/1  "w=ABV"
  dp3 value/1 -> Derivative/1
  Constant/1 -> Product/1
  Saturation/1 -> Product/2

== system simulation model/ESU/fuel subsystem ==
  Wf : Inport
  Bfuel : Constant  Value=Bf
  Demux1 : Demux  Outputs=5
  Derivative : Derivative
  Product : Product
  Saturation : Saturate  UpperLimit=0.25  LowerLimit=-0.25
  DNgf : Outport
  DNpf : Outport  Port=2
  DP4f : Outport  Port=3
  DP45f : Outport  Port=4
  DT45f : Outport  Port=5
  wires:
  Product/1 -> Demux1/1
  Bfuel/1 -> Product/1
  Wf/1 -> Derivative/1
  Demux1/4 -> DP45f/1
  Demux1/1 -> DNgf/1  "wa"
  Demux1/2 -> DNpf/1
  Demux1/3 -> DP4f/1
  Demux1/5 -> DT45f/1
  Derivative/1 -> Saturation/1  "WF"
  Saturation/1 -> Product/2

== system simulation model/ESU/propeller angle subsystem ==
  prop angle : Inport
  Constant1 : Constant  Value=Bp
  Derivative : Derivative
  Product1 : Product
  Saturation : Saturate  UpperLimit=0.25  LowerLimit=-0.25
  dNp PROP : Outport
  wires:
  prop angle/1 -> Derivative/1
  Constant1/1 -> Product1/1
  Derivative/1 -> Saturation/1  "angle"
  Product1/1 -> dNp PROP/1
  Saturation/1 -> Product1/2

== system simulation model/ESU/variable geometry subsystem ==
  "VSV agle " : Inport
  Constant : Constant  Value=Bv
  Demux1 : Demux  Outputs=2
  Derivative : Derivative
  Product : Product
  Saturation : Saturate  UpperLimit=0.25  LowerLimit=-0.25
  Dngv : Outport
  DP3v : Outport  Port=2
  wires:
  Constant/1 -> Product/1
  "VSV agle "/1 -> Derivative/1
  Product/1 -> Demux1/1
  Demux1/2 -> DP3v/1
  Demux1/1 -> Dngv/1
  Derivative/1 -> Saturation/1  "VG"
  Saturation/1 -> Product/2

== system simulation model/ECU / FMV controller/10 value average ==
  Input : Inport
  Add1 : Sum  Inputs=++++++++++
  Constant3 : Constant  Value=10
  Delay : Delay  DelayLength=1  InitialCondition=optimal_rotation
  Delay1 : Delay  InitialCondition=optimal_rotation
  Delay2 : Delay  DelayLength=3  InitialCondition=optimal_rotation
  Delay3 : Delay  DelayLength=4  InitialCondition=optimal_rotation
  Delay4 : Delay  DelayLength=5  InitialCondition=optimal_rotation
  Delay5 : Delay  DelayLength=6  InitialCondition=optimal_rotation
  Delay6 : Delay  DelayLength=7  InitialCondition=optimal_rotation
  Delay7 : Delay  DelayLength=8  InitialCondition=optimal_rotation
  Delay8 : Delay  DelayLength=9  InitialCondition=optimal_rotation
  Divide : Product  Inputs=*/
  Output : Outport
  wires:
  Input/1 -> Delay8/1, Delay7/1, Delay6/1, Delay5/1, Delay4/1, Delay3/1, Delay2/1, Delay1/1, Delay/1, Add1/1
  Delay8/1 -> Add1/10
  Delay2/1 -> Add1/4
  Constant3/1 -> Divide/2
  Add1/1 -> Divide/1
  Divide/1 -> Output/1
  Delay7/1 -> Add1/9
  Delay3/1 -> Add1/5
  Delay6/1 -> Add1/8
  Delay5/1 -> Add1/7
  Delay4/1 -> Add1/6
  Delay/1 -> Add1/2
  Delay1/1 -> Add1/3

== system simulation model/ECU /Ng speed limiters/Safe switch ==
  In1 : Inport
  Add1 : Sum
  Delay : Delay  DelayLength=1
  OFF : Constant  Value=0
  ON : Constant
  Switch1 : Switch  Criteria=u2 > Threshold  Threshold=10  SaturateOnIntegerOverflow=off  InputSameDT=off
  min 0 : Saturate  UpperLimit=100  LowerLimit=0
  Out1 : Outport
  wires:
  ON/1 -> Switch1/1
  Delay/1 -> Add1/2
  Add1/1 -> min 0/1
  Switch1/1 -> Out1/1
  min 0/1 -> Switch1/2, Delay/1
  OFF/1 -> Switch1/3
  In1/1 -> Add1/1

== system simulation model/ECU /No speed limiters/Safe switch ==
  In1 : Inport
  Add1 : Sum
  Delay : Delay  DelayLength=1
  OFF : Constant  Value=0
  ON : Constant
  Switch1 : Switch  Criteria=u2 > Threshold  Threshold=10  SaturateOnIntegerOverflow=off  InputSameDT=off
  min 0 : Saturate  UpperLimit=100  LowerLimit=0
  No to FBV : Outport
  wires:
  ON/1 -> Switch1/1
  Delay/1 -> Add1/2
  Add1/1 -> min 0/1
  Switch1/1 -> No to FBV/1
  min 0/1 -> Switch1/2, Delay/1
  OFF/1 -> Switch1/3
  In1/1 -> Add1/1

== system simulation model/ECU /Np speed limiters/Safe switch ==
  In1 : Inport
  Add1 : Sum
  Delay : Delay  DelayLength=1
  OFF : Constant  Value=0
  ON : Constant
  Switch1 : Switch  Criteria=u2 > Threshold  Threshold=10  SaturateOnIntegerOverflow=off  InputSameDT=off
  min 0 : Saturate  UpperLimit=100  LowerLimit=0
  Np to SOV : Outport
  wires:
  ON/1 -> Switch1/1
  Delay/1 -> Add1/2
  Add1/1 -> min 0/1
  Switch1/1 -> Np to SOV/1
  min 0/1 -> Switch1/2, Delay/1
  OFF/1 -> Switch1/3
  In1/1 -> Add1/1

== system simulation model/ECU /P3t//P2t limiter/Safe switch ==
  In1 : Inport
  Add1 : Sum
  Delay : Delay  DelayLength=1
  OFF : Constant  Value=0
  ON : Constant
  Switch1 : Switch  Criteria=u2 > Threshold  Threshold=10  SaturateOnIntegerOverflow=off  InputSameDT=off
  min 0 : Saturate  UpperLimit=100  LowerLimit=0
  P3t/P2t to ABV : Outport
  wires:
  ON/1 -> Switch1/1
  Delay/1 -> Add1/2
  Add1/1 -> min 0/1
  Switch1/1 -> P3t/P2t to ABV/1
  min 0/1 -> Switch1/2, Delay/1
  OFF/1 -> Switch1/3
  In1/1 -> Add1/1

== system simulation model/ECU /PCV+FBV actuator/angle to % ==
  angle : Inport
  Add : Sum  Inputs=+-
  Add1 : Sum
  Constant : Constant  Value=a_prop
  Constant1 : Constant
  Divide : Product  Inputs=*/
  prop angle% : Outport
  wires:
  Add/1 -> Divide/1
  Constant/1 -> Divide/2, Add/2
  angle/1 -> Add/1
  Divide/1 -> Add1/1
  Add1/1 -> prop angle%/1
  Constant1/1 -> Add1/2

== system simulation model/ECU /T45t limiter/Safe switch ==
  In1 : Inport
  Add1 : Sum
  Delay : Delay  DelayLength=1
  OFF : Constant  Value=0
  ON : Constant
  Switch1 : Switch  Criteria=u2 > Threshold  Threshold=10  SaturateOnIntegerOverflow=off  InputSameDT=off
  min 0 : Saturate  UpperLimit=100  LowerLimit=0
  T45t to SOV : Outport
  wires:
  ON/1 -> Switch1/1
  Delay/1 -> Add1/2
  Add1/1 -> min 0/1
  Switch1/1 -> T45t to SOV/1
  min 0/1 -> Switch1/2, Delay/1
  OFF/1 -> Switch1/3
  In1/1 -> Add1/1

== system simulation model/ECU /Torque limiters/Safe switch ==
  In1 : Inport
  Add1 : Sum
  Delay : Delay  DelayLength=1
  OFF : Constant  Value=0
  ON : Constant
  Switch1 : Switch  Criteria=u2 > Threshold  Threshold=10  SaturateOnIntegerOverflow=off  InputSameDT=off
  min 0 : Saturate  UpperLimit=100  LowerLimit=0
  Torque to SOV : Outport
  wires:
  ON/1 -> Switch1/1
  Delay/1 -> Add1/2
  Add1/1 -> min 0/1
  Switch1/1 -> Torque to SOV/1
  min 0/1 -> Switch1/2, Delay/1
  OFF/1 -> Switch1/3
  In1/1 -> Add1/1

== system simulation model/ECU /VG actuator/angle to angle % ==
  ange deg : Inport
  Add : Sum
  Constant : Constant  Value=20
  Constant1 : Constant  Value=30
  Divide : Product  Inputs=*/
  angle % : Outport
  wires:
  Constant1/1 -> Divide/2
  ange deg/1 -> Add/1
  Divide/1 -> angle %/1
  Constant/1 -> Add/2
  Add/1 -> Divide/1

== system simulation model/ECU /VG controler/10 value average ==
  Input : Inport
  Add1 : Sum  Inputs=++++++++++
  Constant3 : Constant  Value=10
  Delay : Delay  DelayLength=1  InitialCondition=0
  Delay1 : Delay  InitialCondition=0
  Delay2 : Delay  DelayLength=3  InitialCondition=0
  Delay3 : Delay  DelayLength=4  InitialCondition=0
  Delay4 : Delay  DelayLength=5  InitialCondition=0
  Delay5 : Delay  DelayLength=6  InitialCondition=0
  Delay6 : Delay  DelayLength=7  InitialCondition=0
  Delay7 : Delay  DelayLength=8  InitialCondition=0
  Delay8 : Delay  DelayLength=9  InitialCondition=0
  Divide : Product  Inputs=*/
  Output : Outport
  wires:
  Input/1 -> Delay8/1, Delay7/1, Delay6/1, Delay5/1, Delay4/1, Delay3/1, Delay2/1, Delay1/1, Delay/1, Add1/1
  Delay8/1 -> Add1/10
  Delay2/1 -> Add1/4
  Constant3/1 -> Divide/2
  Add1/1 -> Divide/1
  Divide/1 -> Output/1
  Delay7/1 -> Add1/9
  Delay3/1 -> Add1/5
  Delay6/1 -> Add1/8
  Delay5/1 -> Add1/7
  Delay4/1 -> Add1/6
  Delay/1 -> Add1/2
  Delay1/1 -> Add1/3

== matlab function simulation model/ESU/Main subsystem/MATLAB Function1 ==
  data: u input; y output; A input
function y = fcn(u,A)
starter=max(abs(u));
maxer=starter;
[x]=find(abs(u)==maxer,1,"first");
k= x(1,1);
i=0;
while (i<1)
    u=u+A*u;
    u=u+A*u;
    maxer= abs((abs(u(k))-starter))/(starter+0.1);
    i=i+1;
end
    y=u;

== matlab function simulation model/ECU / FMV controller/FMV controller ==
  data: dP3P2 input; dT45 input; y output
function y = fcn(dP3P2,dT45)
u=max(dP3P2,dT45);
y = u;

== matlab function simulation model/ECU /T45t limiter/T45 VOTER ==
  data: u input; y output
function y = fcn(u)
u=sort(u);
y = (u(2)+u(3)+u(4))/3;
